simulink model "blink"  (R2016b)
settings: Solver=FixedStepDiscrete  StartTime=0.0  StopTime=120  RelTol=1e-3
libraries: simulink x2, dspswit3 x1, dspstat3 x1
settings Model: Creator=FWWALSH  LastModifiedBy=Home

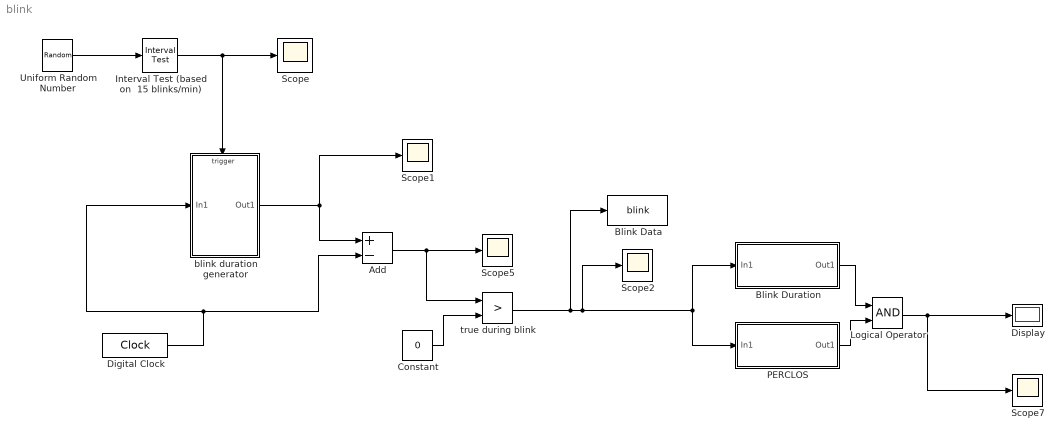
== system blink ==
  Add : Sum  Inputs=+-
  "Blink Data " : ToWorkspace  VariableName=blink  SaveFormat=Timeseries  SampleTime=-1
  "Blink Duration " : Subsystem
  Constant : Constant  Value=0
  Digital Clock : DigitalClock  SampleTime=.1
  Display : Display
  Interval Test (based on  15 blinks/min) : simulink/Logic and Bit Operations/Interval Test  IntervalClosedRight=on  uplimit=0.0025  IntervalClosedLeft=on  lowlimit=0  OutDataTypeStr=boolean
  Logical Operator : Logic  AllPortsSameDT=off  OutDataTypeStr=boolean
  PERCLOS : Subsystem
  Scope{,1..2,5,7} (5 alike) : Scope
  Uniform Random Number : UniformRandomNumber  Minimum=0  Seed=10  SampleTime=0.01
  blink duration generator : Subsystem
  true during blink : RelationalOperator  Operator=>  OutDataTypeStr=boolean  RndMeth=Simplest
  wires:
  blink duration generator/1(Out1) -> Add/1, Scope1/1
  Add/1 -> true during blink/1, Scope5/1
  Interval Test (based on  15 blinks/min)/1 -> Scope/1, blink duration generator/Trigger
  Constant/1 -> true during blink/2
  Uniform Random Number/1 -> Interval Test (based on  15 blinks/min)/1
  Logical Operator/1 -> Display/1, Scope7/1
  Digital Clock/1 -> blink duration generator/1(In1), Add/2
  true during blink/1 -> "Blink Duration "/1(In1), PERCLOS/1(In1), Scope2/1, "Blink Data "/1
  PERCLOS/1(Out1) -> Logical Operator/2
  "Blink Duration "/1(Out1) -> Logical Operator/1

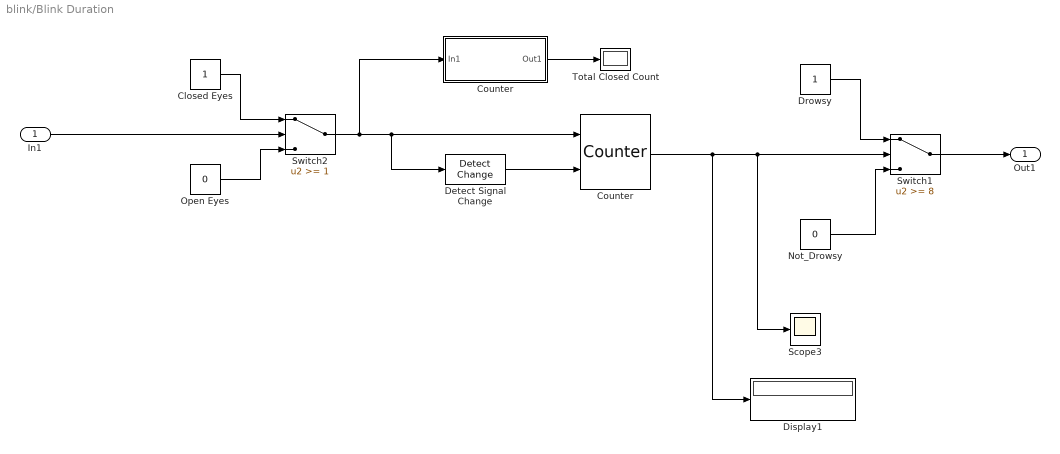
== system blink/Blink Duration  ==
  In1 : Inport
  Closed Eyes : Constant
  Counter : dspswit3/Counter  Direction=Up  CountEvent=Non-zero sample  CounterSize=User defined  MaxCount=25  InitialCount=0  Output=Count  HitValue=32  ResetInput=on  SamplesPerFrame=1  Ts=1  CntDtype=double  HitDtype=Logical
  "Counter " : Subsystem  TreatAsAtomicUnit=on
  Detect Signal Change : simulink/Logic and Bit Operations/Detect Change  vinit=0  OutDataTypeStr=boolean
  Display1 : Display
  Drowsy : Constant
  Not_Drowsy : Constant  Value=0
  Open Eyes : Constant  Value=0
  Scope3 : Scope
  Switch1 : Switch  Threshold=8
  Switch2 : Switch  Threshold=1
  Total Closed Count : Display
  Out1 : Outport
  wires:
  Not_Drowsy/1 -> Switch1/3
  Drowsy/1 -> Switch1/1
  Switch1/1 -> Out1/1
  Open Eyes/1 -> Switch2/3
  Closed Eyes/1 -> Switch2/1
  In1/1 -> Switch2/2
  Counter/1 -> Display1/1, Scope3/1, Switch1/2
  Detect Signal Change/1 -> Counter/2
  "Counter "/1(Out1) -> Total Closed Count/1
  Switch2/1 -> Counter/1, Detect Signal Change/1, "Counter "/1(In1)

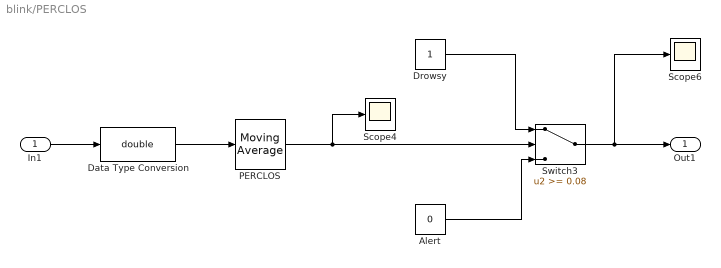
== system blink/PERCLOS ==
  In1 : Inport
  "Alert " : Constant  Value=0
  Data Type Conversion : DataTypeConversion  OutDataTypeStr=double
  "Drowsy " : Constant
  PERCLOS : dspstat3/Moving Average  Method=Sliding window  SpecifyWindowLength=on  WindowLength=3000  ForgettingFactor=0.9  SimulateUsing=Code generation
  Scope4 : Scope
  Scope6 : Scope
  Switch3 : Switch  Threshold=0.08
  Out1 : Outport
  wires:
  Data Type Conversion/1 -> PERCLOS/1
  In1/1 -> Data Type Conversion/1
  PERCLOS/1 -> Switch3/2, Scope4/1
  "Alert "/1 -> Switch3/3
  "Drowsy "/1 -> Switch3/1
  Switch3/1 -> Out1/1, Scope6/1

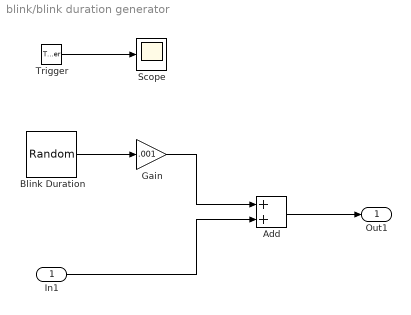
== system blink/blink duration generator ==
  In1 : Inport
  Trigger : TriggerPort  VariantControl=Variant  ShowOutputPort=on  PortDimensions=1
  Add : Sum
  Blink Duration : RandomNumber  Mean=250  Variance=200
  Gain : Gain  Gain=.001
  Scope : Scope
  Out1 : Outport
  wires:
  Blink Duration/1 -> Gain/1
  Trigger/1 -> Scope/1
  In1/1 -> Add/2
  Add/1 -> Out1/1
  Gain/1 -> Add/1

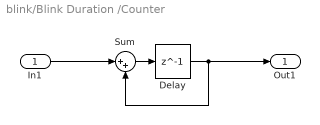
== system blink/Blink Duration /Counter  ==
  In1 : Inport
  Delay : Delay  DelayLength=1  InitialCondition=0
  Sum : Sum  Inputs=|++
  Out1 : Outport
  wires:
  Sum/1 -> Delay/1
  Delay/1 -> Out1/1, Sum/2
  In1/1 -> Sum/1
